simulink model "Quanser_AERO_Simulation_2020b"  (R2020b)
settings: Solver=ode45  StartTime=0.0  StopTime=2*sim_time  FixedStep=0.01  RelTol=1e-3
InitFcn:
  | % Run simulation parameters
  | quanser_AERO_sim_params;
model workspace (MAT data in the model file):
  a = Simulink.Parameter
  a.Value = 1.15
  a.DataType = 'auto'
  a.Dimensions = [1 1]
  a_a = Simulink.Parameter
  a_a.Value = 0.043381
  a_a.DataType = 'auto'
  a_a.Dimensions = [1 1]
  b = Simulink.Parameter
  b.Value = 0.2847
  b.DataType = 'auto'
  b.Dimensions = [1 1]
  b_b = Simulink.Parameter
  b_b.Value = 0.005
  b_b.DataType = 'auto'
  b_b.Dimensions = [1 1]
  c = Simulink.Parameter
  c.Value = 0.53573
  c.DataType = 'auto'
  c.Dimensions = [1 1]
  c_c = Simulink.Parameter
  c_c.Value = 0.005
  c_c.DataType = 'auto'
  c_c.Dimensions = [1 1]
  d = Simulink.Parameter
  d.Value = 0.0071058
  d.DataType = 'auto'
  d.Dimensions = [1 1]
  d_d = Simulink.Parameter
  d_d.Value = 0
  d_d.DataType = 'auto'
  d_d.Dimensions = [1 1]
  e = Simulink.Parameter
  e.Value = 0.0071
  e.DataType = 'auto'
  e.Dimensions = [1 1]
  f = Simulink.Parameter
  f.Value = 0.05
  f.DataType = 'auto'
  f.Dimensions = [1 1]
  g = Simulink.Parameter
  g.Value = 9.81
  g.DataType = 'auto'
  g.Dimensions = [1 1]
  p_p = Simulink.Parameter
  p_p.Value = 0.0005466
  p_p.DataType = 'auto'
  p_p.Dimensions = [1 1]
  smiData.RigidTransform(1).translation = [75 240 -4.4408920985e-15]
  smiData.RigidTransform(1).angle = 1.57079632679
  smiData.RigidTransform(1).axis = [5.55111512313e-17 1 5.55111512313e-17]
  smiData.RigidTransform(1).ID = 'B[AERO - Fork:1:-:AERO - Arm:1]'
  smiData.RigidTransform(2).translation = [0 0 72.5]
  smiData.RigidTransform(2).angle = 0
  smiData.RigidTransform(2).axis = [0 0 0]
  smiData.RigidTransform(2).ID = 'F[AERO - Fork:1:-:AERO - Arm:1]'
  smiData.RigidTransform(3).translation = [53 0 0]
  smiData.RigidTransform(3).angle = 1.57079632679
  smiData.RigidTransform(3).axis = [0 -1 0]
  smiData.RigidTransform(3).ID = 'B[AERO - Arm:1:-:AERO - Propeller Housing:1]'
  smiData.RigidTransform(4).translation = [-2.67952073108e-14 10 -95.5137103749]
  smiData.RigidTransform(4).angle = 3.14159265359
  smiData.RigidTransform(4).axis = [1 0 0]
  smiData.RigidTransform(4).ID = 'F[AERO - Arm:1:-:AERO - Propeller Housing:1]'
  smiData.RigidTransform(5).translation = [-53 0 0]
  smiData.RigidTransform(5).angle = 3.14159265359
  smiData.RigidTransform(5).axis = [0.707106781187 0 0.707106781187]
  smiData.RigidTransform(5).ID = 'B[AERO - Arm:1:-:AERO - Propeller Housing:2]'
  smiData.RigidTransform(6).translation = [-2.67952073108e-14 10 -95.5137103749]
  smiData.RigidTransform(6).angle = 3.14159265359
  smiData.RigidTransform(6).axis = [1 0 0]
  smiData.RigidTransform(6).ID = 'F[AERO - Arm:1:-:AERO - Propeller Housing:2]'
  smiData.RigidTransform(7).translation = [0 90 0]
  smiData.RigidTransform(7).angle = 2.09439510239
  smiData.RigidTransform(7).axis = [-0.57735026919 -0.57735026919 -0.57735026919]
  smiData.RigidTransform(7).ID = 'B[AERO - Base:1:-:AERO - Fork:1]'
  smiData.RigidTransform(8).translation = [0 -10 -1.83697019872e-15]
  smiData.RigidTransform(8).angle = 1.57079632679
  smiData.RigidTransform(8).axis = [-1 0 0]
  smiData.RigidTransform(8).ID = 'F[AERO - Base:1:-:AERO - Fork:1]'
  smiData.RigidTransform(9).translation = [0 7 0]
  smiData.RigidTransform(9).angle = 1.57079632679
  smiData.RigidTransform(9).axis = [-1 1.5327705937e-16 1.5327705937e-16]
  smiData.RigidTransform(9).ID = 'B[AERO - Propeller Housing:1:-:AERO - Propeller:1]'
  smiData.RigidTransform(10).translation = [0 2 0]
  smiData.RigidTransform(10).angle = 1.6664335536
  smiData.RigidTransform(10).axis = [-0.908660854566 0.295241808844 0.295241808844]
  smiData.RigidTransform(10).ID = 'F[AERO - Propeller Housing:1:-:AERO - Propeller:1]'
  smiData.RigidTransform(11).translation = [0 7 0]
  smiData.RigidTransform(11).angle = 1.57079632679
  smiData.RigidTransform(11).axis = [-1 6.25051204106e-17 6.25051204106e-17]
  smiData.RigidTransform(11).ID = 'B[AERO - Propeller Housing:2:-:AERO - Propeller:2]'
  smiData.RigidTransform(12).translation = [0 2 0]
  smiData.RigidTransform(12).angle = 2.28432867519
  smiData.RigidTransform(12).axis = [-0.456966311669 -0.628960169645 -0.628960169645]
  smiData.RigidTransform(12).ID = 'F[AERO - Propeller Housing:2:-:AERO - Propeller:2]'
  smiData.RigidTransform(13).translation = [-4.21383634609 -51.619496794 8.881784197e-15]
  smiData.RigidTransform(13).angle = 0
  smiData.RigidTransform(13).axis = [0 0 0]
  smiData.RigidTransform(13).ID = 'SixDofRigidTransform[AERO - Base:1]'
  smiData.Solid(1).mass = 2.36460135901
  smiData.Solid(1).CoM = [5.24111117378e-10 37.9532129776 0]
  smiData.Solid(1).MoI = [7187.732483 11870.3385044 7187.73246752]
  smiData.Solid(1).PoI = [0 0 -5.80827271444e-08]
  smiData.Solid(1).color = [0.0196078431373 0.0196078431373 0.0196078431373]
  smiData.Solid(1).opacity = 1
  smiData.Solid(1).ID = 'AERO - Base.ipt_{5B170AF7-4835-771C-6ADF-04BDBD784493}'
  smiData.Solid(2).mass = 0.833057949362
  smiData.Solid(2).CoM = [2.66169728603e-11 94.8876622043 1.47659785864e-12]
  smiData.Solid(2).MoI = [5303.1260885 5291.93963258 10383.1205417]
  smiData.Solid(2).PoI = [-1.78319566538e-10 1.20053300634e-10 2.21603950608e-09]
  smiData.Solid(2).color = [0.0196078431373 0.0196078431373 0.0196078431373]
  smiData.Solid(2).opacity = 1
  smiData.Solid(2).ID = 'AERO - Fork.ipt_{19DEB560-4DA8-F02E-E9C0-369FCF880C44}'
  smiData.Solid(3).mass = 0.268036846773
  smiData.Solid(3).CoM = [1.42171296006e-09 -5.19659809406e-10 0]
  smiData.Solid(3).MoI = [365.292105474 461.18513674 151.85502279]
  smiData.Solid(3).PoI = [9.09494701773e-14 -7.58518581279e-10 0]
  smiData.Solid(3).color = [0.0196078431373 0.0196078431373 0.0196078431373]
  smiData.Solid(3).opacity = 1
  smiData.Solid(3).ID = 'AERO - Arm.ipt_{15B1D815-460D-A329-2F9F-5FB9E93ED37B}'
  smiData.Solid(4).mass = 0.12383177107
  smiData.Solid(4).CoM = [0.00177195297055 5.45503898669 -8.60877968745]
  smiData.Solid(4).MoI = [310.701431452 411.715449483 138.600608927]
  smiData.Solid(4).PoI = [4.84491065682 -0.146839869659 -0.00100363322073]
  smiData.Solid(4).color = [0.0196078431373 0.0196078431373 0.0196078431373]
  smiData.Solid(4).opacity = 1
  smiData.Solid(4).ID = 'AERO - Propeller Housing.ipt_{180F9119-4C93-59E3-A88D-3BA97F46F3C3}'
  smiData.Solid(5).mass = 0.0206425497221
  smiData.Solid(5).CoM = [-1.0654070865e-12 5.09575570658 -2.10819251568e-11]
  smiData.Solid(5).MoI = [13.8216638961 27.2772869122 13.8216638974]
  smiData.Solid(5).PoI = [0 0 -9.39933149128e-14]
  smiData.Solid(5).color = [0.121568627451 0.121568627451 0.705882352941]
  smiData.Solid(5).opacity = 1
  smiData.Solid(5).ID = 'AERO - Propeller.ipt_{54ECD9B7-47A0-F6BB-CE8E-F5BB4731363E}'
  smiData.RevoluteJoint(1).Rz.Pos = 8.54433050095e-10
  smiData.RevoluteJoint(1).ID = '[AERO - Fork:1:-:AERO - Arm:1]'
  smiData.RevoluteJoint(2).Rz.Pos = 176.894023419
  smiData.RevoluteJoint(2).ID = '[AERO - Arm:1:-:AERO - Propeller Housing:1]'
  smiData.RevoluteJoint(3).Rz.Pos = 3.10597658118
  smiData.RevoluteJoint(3).ID = '[AERO - Arm:1:-:AERO - Propeller Housing:2]'
  smiData.RevoluteJoint(4).Rz.Pos = -4.73234748156e-11
  smiData.RevoluteJoint(4).ID = '[AERO - Base:1:-:AERO - Fork:1]'
  smiData.RevoluteJoint(5).Rz.Pos = -5.89066785065e-05
  smiData.RevoluteJoint(5).ID = '[AERO - Propeller Housing:1:-:AERO - Propeller:1]'
  smiData.RevoluteJoint(6).Rz.Pos = -3.64250166753e-05
  smiData.RevoluteJoint(6).ID = '[AERO - Propeller Housing:2:-:AERO - Propeller:2]'
  t_t = Simulink.Parameter
  t_t.Value = 0.0005466
  t_t.DataType = 'auto'
  t_t.Dimensions = [1 1]
  u_lim = Simulink.Parameter
  u_lim.Value = 24
  u_lim.DataType = 'auto'
  u_lim.Dimensions = [1 1]
  y_y = Simulink.Parameter
  y_y.Value = 0.02
  y_y.DataType = 'auto'
  y_y.Dimensions = [1 1]
  z_z = Simulink.Parameter
  z_z.Value = 0.01
  z_z.DataType = 'auto'
  z_z.Dimensions = [1 1]
values from neighbouring files (symbols this model uses):
  model = 1    [quanser_AERO_sim_params.m]
  ts = 0.002    [quanser_AERO_sim_params.m]
undefined symbols (not defined in the file or in its folder): delta, delta_a_range, delta_b_range, delta_c_range, den, dena, denb, dend, ini_cond, K, noise, num, numa, numb, numd, X, Y, Z
libraries: sm_lib x595, nesl_utility x119, simulink x102
(part 1 of 18)
settings Model: DataDictionary=AERO_DigitalTwin.sldd  OrderedModelArguments=off  Creator=garciar1  LastModifiedBy=linesLK
settings ExplorerConfigSet: InternalSimMechanicsExplorerSettings="<ExplorerConfiguration><canonicalview>planar_xy</canonicalview><AnimationSetting><BasePlaybackSpeed>1.0</BasePlaybackSpeed><PlaybackSpeedFactor>1.0</PlaybackSpeedFactor></AnimationSetting><TilePanel><TileInfo><Tiles Columns=\"1\" Count=\"1\" Rows=\"1\"><Column Weight=\"1\"/><Row Weight=\"1\"/><Tile Height=\"1\" Width=\"1\" X=\"0\" Y=\"0\"/></Tiles></TileInfo><SceneInfo><SceneViewer><BGColor><R>0.60000002384185791</R><G>0.60000002384185791</G><B>0.60000002384185791</B></BGColor><Camera><DoPerspective>off</DoPerspective><Position><X>0.606138610969192748</X><Y>0.738169372517540556</Y><Z>0.590514966088055981</Z></Position><Center><X>0.0287883417795668992</X><Y>0.160819103327914742</Y><Z>0.0131646968984300838</Z></Center><Up><X>-0.408248290463863073</X><Y>0.816496580927726145</Y><Z>-0.408248290463863073</Z></Up><ViewLimDist>1</ViewLimDist><YLim>0.238299283981323246</YLim><XLim>0.228027763120059318</XLim></Camera></SceneViewer></SceneInfo></TilePanel><MechEditorPanel><Cameras/><GfxPanelCameraMap/><VideoCreator><PlaybackSpeedRatio>1.0</PlaybackSpeedRatio><FrameRate>30</FrameRate><VideoFormat>Motion JPEG AVI</VideoFormat><FrameSize>auto</FrameSize></VideoCreator></MechEditorPanel></ExplorerConfiguration>"

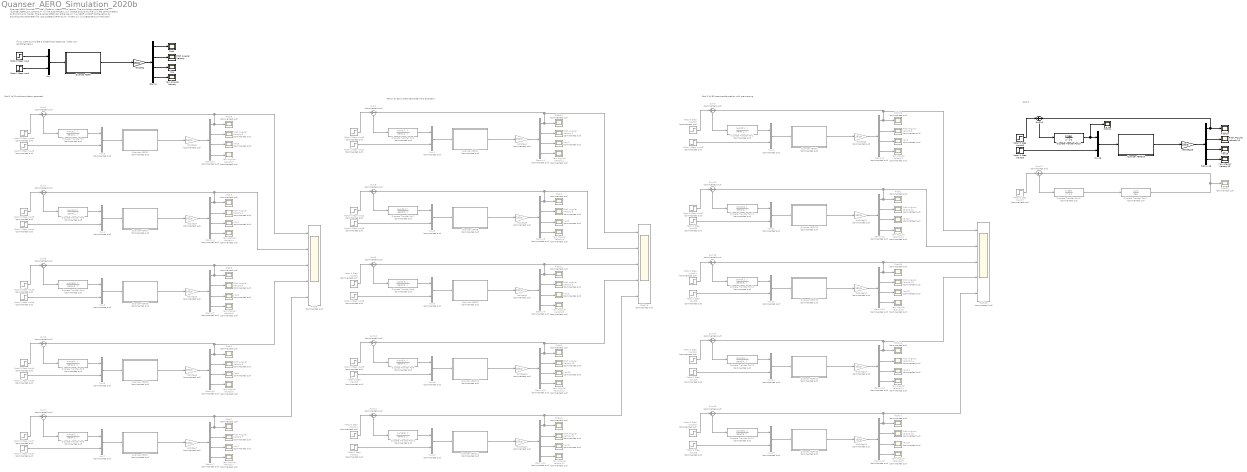
== system Quanser_AERO_Simulation_2020b ==
  note: If you want to simulate a closed-loop response, insert your controller below.
  note: Quanser AERO Simulation Model: Platform Independent Version
      | The simulation parameter file 'quanser_AERO_sim_params.m' will be automatically run, please ensure this file is in the same directory as this Simulink model. The Quanser AERO can either be run in a 1DOF or 2DOF configuration by adjusting the parameter file.
      | Last updated 29-07-21 by Vincent Liu (liuv2@student.unimelb.edu)
  note: Part 2 (a) Simple emulation approach
  note: Part 2 (b) Equivalent zero-order hold approach
  note: Part 2 (c) Bilinear transformation with pre-warping
  note: Part 3
  Demux : Demux
  Demux{1..15} (15 alike) : Demux  Commented=on
  Demux16 : Demux
  Discrete Transfer Fcn : DiscreteTransferFcn  Commented=on  Numerator=numa(1, :)  Denominator=dena(1, :)  SampleTime=delta_a_range(1)
  Discrete Transfer Fcn1 : DiscreteTransferFcn  Commented=on  Numerator=numb(1, :)  Denominator=denb(1, :)  SampleTime=delta_b_range(1)
  Discrete Transfer Fcn10 : DiscreteTransferFcn  Commented=on  Numerator=numb(5, :)  Denominator=denb(5, :)  SampleTime=delta_b_range(5)
  Discrete Transfer Fcn11 : DiscreteTransferFcn  Commented=on  Numerator=numd(2,:)  Denominator=dend(2,:)  SampleTime=delta_c_range(2)
  Discrete Transfer Fcn12 : DiscreteTransferFcn  Commented=on  Numerator=numd(3, :)  Denominator=dend(3, :)  SampleTime=delta_c_range(3)
  Discrete Transfer Fcn13 : DiscreteTransferFcn  Commented=on  Numerator=numd(4, :)  Denominator=dend(4, :)  SampleTime=delta_c_range(4)
  Discrete Transfer Fcn14 : DiscreteTransferFcn  Commented=on  Numerator=numd(5, :)  Denominator=dend(5, :)  SampleTime=delta_c_range(5)
  Discrete Transfer Fcn15 : DiscreteTransferFcn  Numerator=K*den  Denominator=[1 -1 0]  SampleTime=delta
  Discrete Transfer Fcn16 : DiscreteTransferFcn  Commented=on  Numerator=K*den  Denominator=[1 -1 0]  SampleTime=delta
  Discrete Transfer Fcn17 : DiscreteTransferFcn  Commented=on  Numerator=num  Denominator=den  SampleTime=delta
  Discrete Transfer Fcn2 : DiscreteTransferFcn  Commented=on  Numerator=numd(1, :)  Denominator=dend(1, :)  SampleTime=delta_c_range(1)
  Discrete Transfer Fcn3 : DiscreteTransferFcn  Commented=on  Numerator=numa(2,:)  Denominator=dena(2,:)  SampleTime=delta_a_range(2)
  Discrete Transfer Fcn4 : DiscreteTransferFcn  Commented=on  Numerator=numa(3, :)  Denominator=dena(3, :)  SampleTime=delta_a_range(3)
  Discrete Transfer Fcn5 : DiscreteTransferFcn  Commented=on  Numerator=numa(4, :)  Denominator=dena(4, :)  SampleTime=delta_a_range(4)
  Discrete Transfer Fcn6 : DiscreteTransferFcn  Commented=on  Numerator=numa(5, :)  Denominator=dena(5, :)  SampleTime=delta_a_range(5)
  Discrete Transfer Fcn7 : DiscreteTransferFcn  Commented=on  Numerator=numb(2,:)  Denominator=denb(2,:)  SampleTime=delta_b_range(2)
  Discrete Transfer Fcn8 : DiscreteTransferFcn  Commented=on  Numerator=numb(3, :)  Denominator=denb(3, :)  SampleTime=delta_b_range(3)
  Discrete Transfer Fcn9 : DiscreteTransferFcn  Commented=on  Numerator=numb(4, :)  Denominator=denb(4, :)  SampleTime=delta_b_range(4)
  Motor 0 Step Input : Step  After=20  SampleTime=0
  Motor 0 Step Input{1..15,17} (16 alike) : Step  Commented=on  After=10  SampleTime=0
  Motor 0 Step Input16 : Step  After=10  SampleTime=0
  Motor 1 Step Input : Step  After=10  SampleTime=0
  Motor 1 Step Input{1..15} (15 alike) : Step  Commented=on  After=10  SampleTime=0
  Motor 1 Step Input16 : Step  After=10  SampleTime=0
  Mux : Mux  Inputs=2
  Mux{1..15} (15 alike) : Mux  Commented=on  Inputs=2
  Mux16 : Mux  Inputs=2
  Pitch : Scope
  Pitch Angular Velocity : Scope
  Pitch Angular Velocity{1..15} (15 alike) : Scope  Commented=on
  Pitch Angular Velocity16 : Scope
  Pitch{1..7,9..12,14..17,20} (16 alike) : Scope  Commented=on
  Pitch13 : Scope  Commented=on  NumInputPorts=5
  Pitch18 : Scope  Commented=on  NumInputPorts=5
  Pitch19 : Scope
  Pitch21 : Scope
  Pitch8 : Scope  Commented=on  NumInputPorts=5
  Quanser AERO : Subsystem  TreatAsAtomicUnit=on
  Quanser AERO1 : Subsystem  Commented=on  TreatAsAtomicUnit=on
  Quanser AERO10 : Subsystem  Commented=on  TreatAsAtomicUnit=on
  Quanser AERO11 : Subsystem  Commented=on  TreatAsAtomicUnit=on
  Quanser AERO12 : Subsystem  Commented=on  TreatAsAtomicUnit=on
  Quanser AERO13 : Subsystem  Commented=on  TreatAsAtomicUnit=on
  Quanser AERO14 : Subsystem  Commented=on  TreatAsAtomicUnit=on
  Quanser AERO15 : Subsystem  Commented=on  TreatAsAtomicUnit=on
  Quanser AERO16 : Subsystem  TreatAsAtomicUnit=on
  Quanser AERO2 : Subsystem  Commented=on  TreatAsAtomicUnit=on
  Quanser AERO3 : Subsystem  Commented=on  TreatAsAtomicUnit=on
  Quanser AERO4 : Subsystem  Commented=on  TreatAsAtomicUnit=on
  Quanser AERO5 : Subsystem  Commented=on  TreatAsAtomicUnit=on
  Quanser AERO6 : Subsystem  Commented=on  TreatAsAtomicUnit=on
  Quanser AERO7 : Subsystem  Commented=on  TreatAsAtomicUnit=on
  Quanser AERO8 : Subsystem  Commented=on  TreatAsAtomicUnit=on
  Quanser AERO9 : Subsystem  Commented=on  TreatAsAtomicUnit=on
  Sum{1..15,17} (16 alike) : Sum  Commented=on  Inputs=+-
  Sum16 : Sum  Inputs=+-
  Yaw : Scope
  Yaw Angular Velocity : Scope
  Yaw Angular Velocity{1..15} (15 alike) : Scope  Commented=on
  Yaw Angular Velocity16 : Scope
  Yaw{1..15} (15 alike) : Scope  Commented=on
  Yaw16 : Scope
  rad2deg : Gain  Gain=180/pi
  rad2deg{1..15} (15 alike) : Gain  Commented=on  Gain=180/pi
  rad2deg16 : Gain  Gain=180/pi
  wires:
  Demux/3 -> Yaw/1
  Demux/2 -> Pitch Angular Velocity/1
  Demux/4 -> Yaw Angular Velocity/1
  Mux/1 -> Quanser AERO/1(u)  "[V0; V1]"
  rad2deg/1 -> Demux/1
  Quanser AERO/1(x) -> rad2deg/1  "[theta; theta_d; psi; psi_d]"
  Motor 1 Step Input/1 -> Mux/2
  Motor 0 Step Input/1 -> Mux/1
  Demux/1 -> Pitch/1
  rad2deg2/1 -> Demux3/1
  Demux3/1 -> Pitch5/1, Pitch8/1, Sum2/2  "Delta = 0.045"
  Demux3/4 -> Yaw Angular Velocity3/1
  Demux3/3 -> Yaw3/1
  Demux3/2 -> Pitch Angular Velocity3/1
  Motor 1 Step Input3/1 -> Mux3/2
  Quanser AERO3/1(x) -> rad2deg2/1  "[theta; theta_d; psi; psi_d]"
  Mux3/1 -> Quanser AERO3/1(u)  "[V0; V1]"
  Discrete Transfer Fcn/1 -> Mux3/1
  Motor 0 Step Input5/1 -> Sum2/1
  Sum2/1 -> Discrete Transfer Fcn/1
  Mux4/1 -> Quanser AERO4/1(u)  "[V0; V1]"
  Demux4/3 -> Yaw4/1
  Quanser AERO4/1(x) -> rad2deg4/1  "[theta; theta_d; psi; psi_d]"
  Motor 1 Step Input4/1 -> Mux4/2
  Demux4/1 -> Pitch8/2, Sum4/2, Pitch3/1  "Delta = 0.0475"
  rad2deg4/1 -> Demux4/1
  Sum4/1 -> Discrete Transfer Fcn3/1
  Demux4/4 -> Yaw Angular Velocity4/1
  Demux4/2 -> Pitch Angular Velocity4/1
  Motor 0 Step Input3/1 -> Sum4/1
  Discrete Transfer Fcn3/1 -> Mux4/1
  Demux5/3 -> Yaw5/1
  Sum6/1 -> Discrete Transfer Fcn5/1
  Demux6/3 -> Yaw6/1
  rad2deg5/1 -> Demux5/1
  Mux5/1 -> Quanser AERO5/1(u)  "[V0; V1]"
  Motor 0 Step Input4/1 -> Sum6/1
  Quanser AERO5/1(x) -> rad2deg5/1  "[theta; theta_d; psi; psi_d]"
  Demux5/2 -> Pitch Angular Velocity5/1
  Motor 0 Step Input6/1 -> Sum5/1
  Demux5/4 -> Yaw Angular Velocity5/1
  Discrete Transfer Fcn4/1 -> Mux5/1
  Motor 1 Step Input6/1 -> Mux6/2
  Demux5/1 -> Pitch6/1, Sum5/2, Pitch8/3  "Delta = 0.05"
  Sum5/1 -> Discrete Transfer Fcn4/1
  Mux6/1 -> Quanser AERO6/1(u)  "[V0; V1]"
  Quanser AERO6/1(x) -> rad2deg6/1  "[theta; theta_d; psi; psi_d]"
  Motor 1 Step Input5/1 -> Mux5/2
  Demux6/2 -> Pitch Angular Velocity6/1
  Demux6/4 -> Yaw Angular Velocity6/1
  Discrete Transfer Fcn5/1 -> Mux6/1
  rad2deg6/1 -> Demux6/1
  Demux6/1 -> Pitch4/1, Pitch8/4, Sum6/2  "Delta = 0.0525"
  Mux7/1 -> Quanser AERO7/1(u)  "[V0; V1]"
  Motor 1 Step Input7/1 -> Mux7/2
  rad2deg7/1 -> Demux7/1
  Demux7/4 -> Yaw Angular Velocity7/1
  Demux7/3 -> Yaw7/1
  Motor 0 Step Input7/1 -> Sum7/1
  Discrete Transfer Fcn6/1 -> Mux7/1
  Quanser AERO7/1(x) -> rad2deg7/1  "[theta; theta_d; psi; psi_d]"
  Demux7/2 -> Pitch Angular Velocity7/1
  Sum7/1 -> Discrete Transfer Fcn6/1
  Demux7/1 -> Pitch7/1, Pitch8/5, Sum7/2  "Delta = 0.055"
  Motor 1 Step Input10/1 -> Mux10/2
  Demux11/1 -> Pitch12/1, Pitch13/5, Sum11/2  "Delta = 0.0475"
  Demux1/4 -> Yaw Angular Velocity1/1
  Demux10/4 -> Yaw Angular Velocity10/1
  rad2deg11/1 -> Demux11/1
  rad2deg8/1 -> Demux8/1
  Demux8/4 -> Yaw Angular Velocity8/1
  Discrete Transfer Fcn8/1 -> Mux9/1
  Demux11/2 -> Pitch Angular Velocity11/1
  Motor 0 Step Input11/1 -> Sum11/1
  Demux10/2 -> Pitch Angular Velocity10/1
  Mux10/1 -> Quanser AERO10/1(u)  "[V0; V1]"
  rad2deg9/1 -> Demux9/1
  Discrete Transfer Fcn9/1 -> Mux10/1
  Sum11/1 -> Discrete Transfer Fcn10/1
  Quanser AERO1/1(x) -> rad2deg1/1  "[theta; theta_d; psi; psi_d]"
  Motor 1 Step Input1/1 -> Mux1/2
  Discrete Transfer Fcn7/1 -> Mux8/1
  Demux8/1 -> Pitch13/2, Sum8/2, Pitch1/1  "Delta = 0.04"
  Demux1/3 -> Yaw1/1
  Motor 1 Step Input11/1 -> Mux11/2
  Demux10/1 -> Pitch9/1, Pitch13/4, Sum10/2  "Delta = 0.045"
  Demux9/3 -> Yaw9/1
  Motor 0 Step Input8/1 -> Sum10/1
  Sum9/1 -> Discrete Transfer Fcn8/1
  Sum1/1 -> Discrete Transfer Fcn1/1
  Motor 0 Step Input9/1 -> Sum1/1
  Sum8/1 -> Discrete Transfer Fcn7/1
  Motor 1 Step Input9/1 -> Mux9/2
  Demux1/2 -> Pitch Angular Velocity1/1
  Discrete Transfer Fcn1/1 -> Mux1/1
  Quanser AERO9/1(x) -> rad2deg9/1  "[theta; theta_d; psi; psi_d]"
  Mux1/1 -> Quanser AERO1/1(u)  "[V0; V1]"
  Mux8/1 -> Quanser AERO8/1(u)  "[V0; V1]"
  Quanser AERO8/1(x) -> rad2deg8/1  "[theta; theta_d; psi; psi_d]"
  Demux8/2 -> Pitch Angular Velocity8/1
  Demux1/1 -> Pitch10/1, Pitch13/1, Sum1/2  "Delta = 0.0375"
  Motor 1 Step Input8/1 -> Mux8/2
  Demux9/2 -> Pitch Angular Velocity9/1
  Demux9/4 -> Yaw Angular Velocity9/1
  Motor 0 Step Input10/1 -> Sum9/1
  Mux9/1 -> Quanser AERO9/1(u)  "[V0; V1]"
  Demux9/1 -> Pitch11/1, Sum9/2, Pitch13/3  "Delta = 0.0425"
  Demux8/3 -> Yaw8/1
  Demux11/4 -> Yaw Angular Velocity11/1
  Motor 0 Step Input1/1 -> Sum8/1
  Discrete Transfer Fcn10/1 -> Mux11/1
  Demux11/3 -> Yaw11/1
  rad2deg1/1 -> Demux1/1
  rad2deg10/1 -> Demux10/1
  Demux10/3 -> Yaw10/1
  Mux11/1 -> Quanser AERO11/1(u)  "[V0; V1]"
  Quanser AERO10/1(x) -> rad2deg10/1  "[theta; theta_d; psi; psi_d]"
  Sum10/1 -> Discrete Transfer Fcn9/1
  Quanser AERO11/1(x) -> rad2deg11/1  "[theta; theta_d; psi; psi_d]"
  Motor 1 Step Input14/1 -> Mux14/2
  Demux15/1 -> Pitch17/1, Pitch18/5, Sum15/2  "Delta = 0.055"
  Demux2/4 -> Yaw Angular Velocity2/1
  Demux14/4 -> Yaw Angular Velocity14/1
  rad2deg15/1 -> Demux15/1
  rad2deg12/1 -> Demux12/1
  Demux12/4 -> Yaw Angular Velocity12/1
  Discrete Transfer Fcn12/1 -> Mux13/1
  Demux15/2 -> Pitch Angular Velocity15/1
  Motor 0 Step Input15/1 -> Sum15/1
  Demux14/2 -> Pitch Angular Velocity14/1
  Mux14/1 -> Quanser AERO14/1(u)  "[V0; V1]"
  rad2deg13/1 -> Demux13/1
  Discrete Transfer Fcn13/1 -> Mux14/1
  Sum15/1 -> Discrete Transfer Fcn14/1
  Quanser AERO2/1(x) -> rad2deg3/1  "[theta; theta_d; psi; psi_d]"
  Motor 1 Step Input2/1 -> Mux2/2
  Discrete Transfer Fcn11/1 -> Mux12/1
  Demux12/1 -> Pitch18/2, Sum12/2, Pitch2/1  "Delta = 0.0475"
  Demux2/3 -> Yaw2/1
  Motor 1 Step Input15/1 -> Mux15/2
  Demux14/1 -> Pitch14/1, Pitch18/4, Sum14/2  "Delta = 0.0525"
  Demux13/3 -> Yaw13/1
  Motor 0 Step Input12/1 -> Sum14/1
  Sum13/1 -> Discrete Transfer Fcn12/1
  Sum3/1 -> Discrete Transfer Fcn2/1
  Motor 0 Step Input13/1 -> Sum3/1
  Sum12/1 -> Discrete Transfer Fcn11/1
  Motor 1 Step Input13/1 -> Mux13/2
  Demux2/2 -> Pitch Angular Velocity2/1
  Discrete Transfer Fcn2/1 -> Mux2/1
  Quanser AERO13/1(x) -> rad2deg13/1  "[theta; theta_d; psi; psi_d]"
  Mux2/1 -> Quanser AERO2/1(u)  "[V0; V1]"
  Mux12/1 -> Quanser AERO12/1(u)  "[V0; V1]"
  Quanser AERO12/1(x) -> rad2deg12/1  "[theta; theta_d; psi; psi_d]"
  Demux12/2 -> Pitch Angular Velocity12/1
  Demux2/1 -> Pitch15/1, Pitch18/1, Sum3/2  "Delta = 0.045"
  Motor 1 Step Input12/1 -> Mux12/2
  Demux13/2 -> Pitch Angular Velocity13/1
  Demux13/4 -> Yaw Angular Velocity13/1
  Motor 0 Step Input14/1 -> Sum13/1
  Mux13/1 -> Quanser AERO13/1(u)  "[V0; V1]"
  Demux13/1 -> Pitch16/1, Sum13/2, Pitch18/3  "Delta = 0.05"
  Demux12/3 -> Yaw12/1
  Demux15/4 -> Yaw Angular Velocity15/1
  Motor 0 Step Input2/1 -> Sum12/1
  Discrete Transfer Fcn14/1 -> Mux15/1
  Demux15/3 -> Yaw15/1
  rad2deg3/1 -> Demux2/1
  rad2deg14/1 -> Demux14/1
  Demux14/3 -> Yaw14/1
  Mux15/1 -> Quanser AERO15/1(u)  "[V0; V1]"
  Quanser AERO14/1(x) -> rad2deg14/1  "[theta; theta_d; psi; psi_d]"
  Sum14/1 -> Discrete Transfer Fcn13/1
  Quanser AERO15/1(x) -> rad2deg15/1  "[theta; theta_d; psi; psi_d]"
  rad2deg16/1 -> Demux16/1
  Sum16/1 -> Discrete Transfer Fcn15/1
  Motor 1 Step Input16/1 -> Mux16/2
  Quanser AERO16/1(x) -> rad2deg16/1  "[theta; theta_d; psi; psi_d]"
  Motor 0 Step Input16/1 -> Sum16/1
  Mux16/1 -> Quanser AERO16/1(u)  "[V0; V1]"
  Demux16/2 -> Pitch Angular Velocity16/1
  Discrete Transfer Fcn15/1 -> Pitch21/1, Mux16/1
  Demux16/3 -> Yaw16/1
  Demux16/1 -> Pitch19/1, Sum16/2  "Delta = 0.05"
  Demux16/4 -> Yaw Angular Velocity16/1
  Sum17/1 -> Discrete Transfer Fcn16/1
  Motor 0 Step Input17/1 -> Sum17/1
  Discrete Transfer Fcn16/1 -> Discrete Transfer Fcn17/1
  Discrete Transfer Fcn17/1 -> Pitch20/1, Sum17/2  "Delta = 0.05"

== system Quanser_AERO_Simulation_2020b/Quanser AERO ==
  u : Inport
  Constant : Constant  Value=model
  Demux : Demux  Outputs=2
  Demux1 : Demux  Outputs=2
  Digital Twin : Subsystem
  Input Noise : Subsystem  TreatAsAtomicUnit=on
  Integrator : Integrator  InitialCondition=[ini_cond.theta; ini_cond.theta_dot; ini_cond.psi; ini_cond.psi_dot]
  Measurement Noise : Subsystem  TreatAsAtomicUnit=on
  Quanser AERO System Dynamics : Subsystem  TreatAsAtomicUnit=on
  Rate Transition : RateTransition  OutPortSampleTime=ts
  Rate Transition1 : RateTransition  InitialCondition=[ini_cond.theta; ini_cond.theta_dot; ini_cond.psi; ini_cond.psi_dot]  OutPortSampleTime=ts
  Selector : Selector  InputPortWidth=4  IndexOptions=Index vector (dialog)  Indices=[1 3]  OutputSizes=1
  x : Outport  VectorParamsAs1DForOutWhenUnconnected=off
  wires:
  u/1 -> Rate Transition/1
  Rate Transition/1 -> Input Noise/1(u), Demux/1
  Rate Transition1/1 -> x/1
  Input Noise/1(u_noise) -> Quanser AERO System Dynamics/2(u)
  Measurement Noise/1(x_noise) -> Rate Transition1/1
  Selector/1 -> Demux1/1
  Demux/1 -> Digital Twin/3(thruster_1)
  Demux/2 -> Digital Twin/4(thruster_2)
  Demux1/1 -> Digital Twin/1(theta)
  Demux1/2 -> Digital Twin/2(psi)
  Integrator/1 -> Measurement Noise/1(x), Selector/1, Quanser AERO System Dynamics/1(x)
  Constant/1 -> Quanser AERO System Dynamics/3(model)
  Quanser AERO System Dynamics/1(x_dot) -> Integrator/1

== system Quanser_AERO_Simulation_2020b/Quanser AERO1 ==
  u : Inport
  Constant : Constant  Value=model
  Demux : Demux  Outputs=2
  Demux1 : Demux  Outputs=2
  Digital Twin : Subsystem
  Input Noise : Subsystem  TreatAsAtomicUnit=on
  Integrator : Integrator  InitialCondition=[ini_cond.theta; ini_cond.theta_dot; ini_cond.psi; ini_cond.psi_dot]
  Measurement Noise : Subsystem  TreatAsAtomicUnit=on
  Quanser AERO System Dynamics : Subsystem  TreatAsAtomicUnit=on
  Rate Transition : RateTransition  OutPortSampleTime=ts
  Rate Transition1 : RateTransition  InitialCondition=[ini_cond.theta; ini_cond.theta_dot; ini_cond.psi; ini_cond.psi_dot]  OutPortSampleTime=ts
  Selector : Selector  InputPortWidth=4  IndexOptions=Index vector (dialog)  Indices=[1 3]  OutputSizes=1
  x : Outport  VectorParamsAs1DForOutWhenUnconnected=off
  wires:
  u/1 -> Rate Transition/1
  Rate Transition/1 -> Input Noise/1(u), Demux/1
  Rate Transition1/1 -> x/1
  Input Noise/1(u_noise) -> Quanser AERO System Dynamics/2(u)
  Measurement Noise/1(x_noise) -> Rate Transition1/1
  Selector/1 -> Demux1/1
  Demux/1 -> Digital Twin/3(thruster_1)
  Demux/2 -> Digital Twin/4(thruster_2)
  Demux1/1 -> Digital Twin/1(theta)
  Demux1/2 -> Digital Twin/2(psi)
  Integrator/1 -> Measurement Noise/1(x), Selector/1, Quanser AERO System Dynamics/1(x)
  Constant/1 -> Quanser AERO System Dynamics/3(model)
  Quanser AERO System Dynamics/1(x_dot) -> Integrator/1

== system Quanser_AERO_Simulation_2020b/Quanser AERO10 ==
  u : Inport
  Constant : Constant  Value=model
  Demux : Demux  Outputs=2
  Demux1 : Demux  Outputs=2
  Digital Twin : Subsystem
  Input Noise : Subsystem  TreatAsAtomicUnit=on
  Integrator : Integrator  InitialCondition=[ini_cond.theta; ini_cond.theta_dot; ini_cond.psi; ini_cond.psi_dot]
  Measurement Noise : Subsystem  TreatAsAtomicUnit=on
  Quanser AERO System Dynamics : Subsystem  TreatAsAtomicUnit=on
  Rate Transition : RateTransition  OutPortSampleTime=ts
  Rate Transition1 : RateTransition  InitialCondition=[ini_cond.theta; ini_cond.theta_dot; ini_cond.psi; ini_cond.psi_dot]  OutPortSampleTime=ts
  Selector : Selector  InputPortWidth=4  IndexOptions=Index vector (dialog)  Indices=[1 3]  OutputSizes=1
  x : Outport  VectorParamsAs1DForOutWhenUnconnected=off
  wires:
  u/1 -> Rate Transition/1
  Rate Transition/1 -> Input Noise/1(u), Demux/1
  Rate Transition1/1 -> x/1
  Input Noise/1(u_noise) -> Quanser AERO System Dynamics/2(u)
  Measurement Noise/1(x_noise) -> Rate Transition1/1
  Selector/1 -> Demux1/1
  Demux/1 -> Digital Twin/3(thruster_1)
  Demux/2 -> Digital Twin/4(thruster_2)
  Demux1/1 -> Digital Twin/1(theta)
  Demux1/2 -> Digital Twin/2(psi)
  Integrator/1 -> Measurement Noise/1(x), Selector/1, Quanser AERO System Dynamics/1(x)
  Constant/1 -> Quanser AERO System Dynamics/3(model)
  Quanser AERO System Dynamics/1(x_dot) -> Integrator/1

== system Quanser_AERO_Simulation_2020b/Quanser AERO11 ==
  u : Inport
  Constant : Constant  Value=model
  Demux : Demux  Outputs=2
  Demux1 : Demux  Outputs=2
  Digital Twin : Subsystem
  Input Noise : Subsystem  TreatAsAtomicUnit=on
  Integrator : Integrator  InitialCondition=[ini_cond.theta; ini_cond.theta_dot; ini_cond.psi; ini_cond.psi_dot]
  Measurement Noise : Subsystem  TreatAsAtomicUnit=on
  Quanser AERO System Dynamics : Subsystem  TreatAsAtomicUnit=on
  Rate Transition : RateTransition  OutPortSampleTime=ts
  Rate Transition1 : RateTransition  InitialCondition=[ini_cond.theta; ini_cond.theta_dot; ini_cond.psi; ini_cond.psi_dot]  OutPortSampleTime=ts
  Selector : Selector  InputPortWidth=4  IndexOptions=Index vector (dialog)  Indices=[1 3]  OutputSizes=1
  x : Outport  VectorParamsAs1DForOutWhenUnconnected=off
  wires:
  u/1 -> Rate Transition/1
  Rate Transition/1 -> Input Noise/1(u), Demux/1
  Rate Transition1/1 -> x/1
  Input Noise/1(u_noise) -> Quanser AERO System Dynamics/2(u)
  Measurement Noise/1(x_noise) -> Rate Transition1/1
  Selector/1 -> Demux1/1
  Demux/1 -> Digital Twin/3(thruster_1)
  Demux/2 -> Digital Twin/4(thruster_2)
  Demux1/1 -> Digital Twin/1(theta)
  Demux1/2 -> Digital Twin/2(psi)
  Integrator/1 -> Measurement Noise/1(x), Selector/1, Quanser AERO System Dynamics/1(x)
  Constant/1 -> Quanser AERO System Dynamics/3(model)
  Quanser AERO System Dynamics/1(x_dot) -> Integrator/1

== system Quanser_AERO_Simulation_2020b/Quanser AERO12 ==
  u : Inport
  Constant : Constant  Value=model
  Demux : Demux  Outputs=2
  Demux1 : Demux  Outputs=2
  Digital Twin : Subsystem
  Input Noise : Subsystem  TreatAsAtomicUnit=on
  Integrator : Integrator  InitialCondition=[ini_cond.theta; ini_cond.theta_dot; ini_cond.psi; ini_cond.psi_dot]
  Measurement Noise : Subsystem  TreatAsAtomicUnit=on
  Quanser AERO System Dynamics : Subsystem  TreatAsAtomicUnit=on
  Rate Transition : RateTransition  OutPortSampleTime=ts
  Rate Transition1 : RateTransition  InitialCondition=[ini_cond.theta; ini_cond.theta_dot; ini_cond.psi; ini_cond.psi_dot]  OutPortSampleTime=ts
  Selector : Selector  InputPortWidth=4  IndexOptions=Index vector (dialog)  Indices=[1 3]  OutputSizes=1
  x : Outport  VectorParamsAs1DForOutWhenUnconnected=off
  wires:
  u/1 -> Rate Transition/1
  Rate Transition/1 -> Input Noise/1(u), Demux/1
  Rate Transition1/1 -> x/1
  Input Noise/1(u_noise) -> Quanser AERO System Dynamics/2(u)
  Measurement Noise/1(x_noise) -> Rate Transition1/1
  Selector/1 -> Demux1/1
  Demux/1 -> Digital Twin/3(thruster_1)
  Demux/2 -> Digital Twin/4(thruster_2)
  Demux1/1 -> Digital Twin/1(theta)
  Demux1/2 -> Digital Twin/2(psi)
  Integrator/1 -> Measurement Noise/1(x), Selector/1, Quanser AERO System Dynamics/1(x)
  Constant/1 -> Quanser AERO System Dynamics/3(model)
  Quanser AERO System Dynamics/1(x_dot) -> Integrator/1

== system Quanser_AERO_Simulation_2020b/Quanser AERO13 ==
  u : Inport
  Constant : Constant  Value=model
  Demux : Demux  Outputs=2
  Demux1 : Demux  Outputs=2
  Digital Twin : Subsystem
  Input Noise : Subsystem  TreatAsAtomicUnit=on
  Integrator : Integrator  InitialCondition=[ini_cond.theta; ini_cond.theta_dot; ini_cond.psi; ini_cond.psi_dot]
  Measurement Noise : Subsystem  TreatAsAtomicUnit=on
  Quanser AERO System Dynamics : Subsystem  TreatAsAtomicUnit=on
  Rate Transition : RateTransition  OutPortSampleTime=ts
  Rate Transition1 : RateTransition  InitialCondition=[ini_cond.theta; ini_cond.theta_dot; ini_cond.psi; ini_cond.psi_dot]  OutPortSampleTime=ts
  Selector : Selector  InputPortWidth=4  IndexOptions=Index vector (dialog)  Indices=[1 3]  OutputSizes=1
  x : Outport  VectorParamsAs1DForOutWhenUnconnected=off
  wires:
  u/1 -> Rate Transition/1
  Rate Transition/1 -> Input Noise/1(u), Demux/1
  Rate Transition1/1 -> x/1
  Input Noise/1(u_noise) -> Quanser AERO System Dynamics/2(u)
  Measurement Noise/1(x_noise) -> Rate Transition1/1
  Selector/1 -> Demux1/1
  Demux/1 -> Digital Twin/3(thruster_1)
  Demux/2 -> Digital Twin/4(thruster_2)
  Demux1/1 -> Digital Twin/1(theta)
  Demux1/2 -> Digital Twin/2(psi)
  Integrator/1 -> Measurement Noise/1(x), Selector/1, Quanser AERO System Dynamics/1(x)
  Constant/1 -> Quanser AERO System Dynamics/3(model)
  Quanser AERO System Dynamics/1(x_dot) -> Integrator/1

== system Quanser_AERO_Simulation_2020b/Quanser AERO14 ==
  u : Inport
  Constant : Constant  Value=model
  Demux : Demux  Outputs=2
  Demux1 : Demux  Outputs=2
  Digital Twin : Subsystem
  Input Noise : Subsystem  TreatAsAtomicUnit=on
  Integrator : Integrator  InitialCondition=[ini_cond.theta; ini_cond.theta_dot; ini_cond.psi; ini_cond.psi_dot]
  Measurement Noise : Subsystem  TreatAsAtomicUnit=on
  Quanser AERO System Dynamics : Subsystem  TreatAsAtomicUnit=on
  Rate Transition : RateTransition  OutPortSampleTime=ts
  Rate Transition1 : RateTransition  InitialCondition=[ini_cond.theta; ini_cond.theta_dot; ini_cond.psi; ini_cond.psi_dot]  OutPortSampleTime=ts
  Selector : Selector  InputPortWidth=4  IndexOptions=Index vector (dialog)  Indices=[1 3]  OutputSizes=1
  x : Outport  VectorParamsAs1DForOutWhenUnconnected=off
  wires:
  u/1 -> Rate Transition/1
  Rate Transition/1 -> Input Noise/1(u), Demux/1
  Rate Transition1/1 -> x/1
  Input Noise/1(u_noise) -> Quanser AERO System Dynamics/2(u)
  Measurement Noise/1(x_noise) -> Rate Transition1/1
  Selector/1 -> Demux1/1
  Demux/1 -> Digital Twin/3(thruster_1)
  Demux/2 -> Digital Twin/4(thruster_2)
  Demux1/1 -> Digital Twin/1(theta)
  Demux1/2 -> Digital Twin/2(psi)
  Integrator/1 -> Measurement Noise/1(x), Selector/1, Quanser AERO System Dynamics/1(x)
  Constant/1 -> Quanser AERO System Dynamics/3(model)
  Quanser AERO System Dynamics/1(x_dot) -> Integrator/1

== system Quanser_AERO_Simulation_2020b/Quanser AERO15 ==
  u : Inport
  Constant : Constant  Value=model
  Demux : Demux  Outputs=2
  Demux1 : Demux  Outputs=2
  Digital Twin : Subsystem
  Input Noise : Subsystem  TreatAsAtomicUnit=on
  Integrator : Integrator  InitialCondition=[ini_cond.theta; ini_cond.theta_dot; ini_cond.psi; ini_cond.psi_dot]
  Measurement Noise : Subsystem  TreatAsAtomicUnit=on
  Quanser AERO System Dynamics : Subsystem  TreatAsAtomicUnit=on
  Rate Transition : RateTransition  OutPortSampleTime=ts
  Rate Transition1 : RateTransition  InitialCondition=[ini_cond.theta; ini_cond.theta_dot; ini_cond.psi; ini_cond.psi_dot]  OutPortSampleTime=ts
  Selector : Selector  InputPortWidth=4  IndexOptions=Index vector (dialog)  Indices=[1 3]  OutputSizes=1
  x : Outport  VectorParamsAs1DForOutWhenUnconnected=off
  wires:
  u/1 -> Rate Transition/1
  Rate Transition/1 -> Input Noise/1(u), Demux/1
  Rate Transition1/1 -> x/1
  Input Noise/1(u_noise) -> Quanser AERO System Dynamics/2(u)
  Measurement Noise/1(x_noise) -> Rate Transition1/1
  Selector/1 -> Demux1/1
  Demux/1 -> Digital Twin/3(thruster_1)
  Demux/2 -> Digital Twin/4(thruster_2)
  Demux1/1 -> Digital Twin/1(theta)
  Demux1/2 -> Digital Twin/2(psi)
  Integrator/1 -> Measurement Noise/1(x), Selector/1, Quanser AERO System Dynamics/1(x)
  Constant/1 -> Quanser AERO System Dynamics/3(model)
  Quanser AERO System Dynamics/1(x_dot) -> Integrator/1

== system Quanser_AERO_Simulation_2020b/Quanser AERO16 ==
  u : Inport
  Constant : Constant  Value=model
  Demux : Demux  Outputs=2
  Demux1 : Demux  Outputs=2
  Digital Twin : Subsystem
  Input Noise : Subsystem  TreatAsAtomicUnit=on
  Integrator : Integrator  InitialCondition=[ini_cond.theta; ini_cond.theta_dot; ini_cond.psi; ini_cond.psi_dot]
  Measurement Noise : Subsystem  TreatAsAtomicUnit=on
  Quanser AERO System Dynamics : Subsystem  TreatAsAtomicUnit=on
  Rate Transition : RateTransition  OutPortSampleTime=ts
  Rate Transition1 : RateTransition  InitialCondition=[ini_cond.theta; ini_cond.theta_dot; ini_cond.psi; ini_cond.psi_dot]  OutPortSampleTime=ts
  Selector : Selector  InputPortWidth=4  IndexOptions=Index vector (dialog)  Indices=[1 3]  OutputSizes=1
  x : Outport  VectorParamsAs1DForOutWhenUnconnected=off
  wires:
  u/1 -> Rate Transition/1
  Rate Transition/1 -> Input Noise/1(u), Demux/1
  Rate Transition1/1 -> x/1
  Input Noise/1(u_noise) -> Quanser AERO System Dynamics/2(u)
  Measurement Noise/1(x_noise) -> Rate Transition1/1
  Selector/1 -> Demux1/1
  Demux/1 -> Digital Twin/3(thruster_1)
  Demux/2 -> Digital Twin/4(thruster_2)
  Demux1/1 -> Digital Twin/1(theta)
  Demux1/2 -> Digital Twin/2(psi)
  Integrator/1 -> Measurement Noise/1(x), Selector/1, Quanser AERO System Dynamics/1(x)
  Constant/1 -> Quanser AERO System Dynamics/3(model)
  Quanser AERO System Dynamics/1(x_dot) -> Integrator/1

== system Quanser_AERO_Simulation_2020b/Quanser AERO2 ==
  u : Inport
  Constant : Constant  Value=model
  Demux : Demux  Outputs=2
  Demux1 : Demux  Outputs=2
  Digital Twin : Subsystem
  Input Noise : Subsystem  TreatAsAtomicUnit=on
  Integrator : Integrator  InitialCondition=[ini_cond.theta; ini_cond.theta_dot; ini_cond.psi; ini_cond.psi_dot]
  Measurement Noise : Subsystem  TreatAsAtomicUnit=on
  Quanser AERO System Dynamics : Subsystem  TreatAsAtomicUnit=on
  Rate Transition : RateTransition  OutPortSampleTime=ts
  Rate Transition1 : RateTransition  InitialCondition=[ini_cond.theta; ini_cond.theta_dot; ini_cond.psi; ini_cond.psi_dot]  OutPortSampleTime=ts
  Selector : Selector  InputPortWidth=4  IndexOptions=Index vector (dialog)  Indices=[1 3]  OutputSizes=1
  x : Outport  VectorParamsAs1DForOutWhenUnconnected=off
  wires:
  u/1 -> Rate Transition/1
  Rate Transition/1 -> Input Noise/1(u), Demux/1
  Rate Transition1/1 -> x/1
  Input Noise/1(u_noise) -> Quanser AERO System Dynamics/2(u)
  Measurement Noise/1(x_noise) -> Rate Transition1/1
  Selector/1 -> Demux1/1
  Demux/1 -> Digital Twin/3(thruster_1)
  Demux/2 -> Digital Twin/4(thruster_2)
  Demux1/1 -> Digital Twin/1(theta)
  Demux1/2 -> Digital Twin/2(psi)
  Integrator/1 -> Measurement Noise/1(x), Selector/1, Quanser AERO System Dynamics/1(x)
  Constant/1 -> Quanser AERO System Dynamics/3(model)
  Quanser AERO System Dynamics/1(x_dot) -> Integrator/1

== system Quanser_AERO_Simulation_2020b/Quanser AERO3 ==
  u : Inport
  Constant : Constant  Value=model
  Demux : Demux  Outputs=2
  Demux1 : Demux  Outputs=2
  Digital Twin : Subsystem
  Input Noise : Subsystem  TreatAsAtomicUnit=on
  Integrator : Integrator  InitialCondition=[ini_cond.theta; ini_cond.theta_dot; ini_cond.psi; ini_cond.psi_dot]
  Measurement Noise : Subsystem  TreatAsAtomicUnit=on
  Quanser AERO System Dynamics : Subsystem  TreatAsAtomicUnit=on
  Rate Transition : RateTransition  OutPortSampleTime=ts
  Rate Transition1 : RateTransition  InitialCondition=[ini_cond.theta; ini_cond.theta_dot; ini_cond.psi; ini_cond.psi_dot]  OutPortSampleTime=ts
  Selector : Selector  InputPortWidth=4  IndexOptions=Index vector (dialog)  Indices=[1 3]  OutputSizes=1
  x : Outport  VectorParamsAs1DForOutWhenUnconnected=off
  wires:
  u/1 -> Rate Transition/1
  Rate Transition/1 -> Input Noise/1(u), Demux/1
  Rate Transition1/1 -> x/1
  Input Noise/1(u_noise) -> Quanser AERO System Dynamics/2(u)
  Measurement Noise/1(x_noise) -> Rate Transition1/1
  Selector/1 -> Demux1/1
  Demux/1 -> Digital Twin/3(thruster_1)
  Demux/2 -> Digital Twin/4(thruster_2)
  Demux1/1 -> Digital Twin/1(theta)
  Demux1/2 -> Digital Twin/2(psi)
  Integrator/1 -> Measurement Noise/1(x), Selector/1, Quanser AERO System Dynamics/1(x)
  Constant/1 -> Quanser AERO System Dynamics/3(model)
  Quanser AERO System Dynamics/1(x_dot) -> Integrator/1

== system Quanser_AERO_Simulation_2020b/Quanser AERO4 ==
  u : Inport
  Constant : Constant  Value=model
  Demux : Demux  Outputs=2
  Demux1 : Demux  Outputs=2
  Digital Twin : Subsystem
  Input Noise : Subsystem  TreatAsAtomicUnit=on
  Integrator : Integrator  InitialCondition=[ini_cond.theta; ini_cond.theta_dot; ini_cond.psi; ini_cond.psi_dot]
  Measurement Noise : Subsystem  TreatAsAtomicUnit=on
  Quanser AERO System Dynamics : Subsystem  TreatAsAtomicUnit=on
  Rate Transition : RateTransition  OutPortSampleTime=ts
  Rate Transition1 : RateTransition  InitialCondition=[ini_cond.theta; ini_cond.theta_dot; ini_cond.psi; ini_cond.psi_dot]  OutPortSampleTime=ts
  Selector : Selector  InputPortWidth=4  IndexOptions=Index vector (dialog)  Indices=[1 3]  OutputSizes=1
  x : Outport  VectorParamsAs1DForOutWhenUnconnected=off
  wires:
  u/1 -> Rate Transition/1
  Rate Transition/1 -> Input Noise/1(u), Demux/1
  Rate Transition1/1 -> x/1
  Input Noise/1(u_noise) -> Quanser AERO System Dynamics/2(u)
  Measurement Noise/1(x_noise) -> Rate Transition1/1
  Selector/1 -> Demux1/1
  Demux/1 -> Digital Twin/3(thruster_1)
  Demux/2 -> Digital Twin/4(thruster_2)
  Demux1/1 -> Digital Twin/1(theta)
  Demux1/2 -> Digital Twin/2(psi)
  Integrator/1 -> Measurement Noise/1(x), Selector/1, Quanser AERO System Dynamics/1(x)
  Constant/1 -> Quanser AERO System Dynamics/3(model)
  Quanser AERO System Dynamics/1(x_dot) -> Integrator/1

== system Quanser_AERO_Simulation_2020b/Quanser AERO5 ==
  u : Inport
  Constant : Constant  Value=model
  Demux : Demux  Outputs=2
  Demux1 : Demux  Outputs=2
  Digital Twin : Subsystem
  Input Noise : Subsystem  TreatAsAtomicUnit=on
  Integrator : Integrator  InitialCondition=[ini_cond.theta; ini_cond.theta_dot; ini_cond.psi; ini_cond.psi_dot]
  Measurement Noise : Subsystem  TreatAsAtomicUnit=on
  Quanser AERO System Dynamics : Subsystem  TreatAsAtomicUnit=on
  Rate Transition : RateTransition  OutPortSampleTime=ts
  Rate Transition1 : RateTransition  InitialCondition=[ini_cond.theta; ini_cond.theta_dot; ini_cond.psi; ini_cond.psi_dot]  OutPortSampleTime=ts
  Selector : Selector  InputPortWidth=4  IndexOptions=Index vector (dialog)  Indices=[1 3]  OutputSizes=1
  x : Outport  VectorParamsAs1DForOutWhenUnconnected=off
  wires:
  u/1 -> Rate Transition/1
  Rate Transition/1 -> Input Noise/1(u), Demux/1
  Rate Transition1/1 -> x/1
  Input Noise/1(u_noise) -> Quanser AERO System Dynamics/2(u)
  Measurement Noise/1(x_noise) -> Rate Transition1/1
  Selector/1 -> Demux1/1
  Demux/1 -> Digital Twin/3(thruster_1)
  Demux/2 -> Digital Twin/4(thruster_2)
  Demux1/1 -> Digital Twin/1(theta)
  Demux1/2 -> Digital Twin/2(psi)
  Integrator/1 -> Measurement Noise/1(x), Selector/1, Quanser AERO System Dynamics/1(x)
  Constant/1 -> Quanser AERO System Dynamics/3(model)
  Quanser AERO System Dynamics/1(x_dot) -> Integrator/1

== system Quanser_AERO_Simulation_2020b/Quanser AERO6 ==
  u : Inport
  Constant : Constant  Value=model
  Demux : Demux  Outputs=2
  Demux1 : Demux  Outputs=2
  Digital Twin : Subsystem
  Input Noise : Subsystem  TreatAsAtomicUnit=on
  Integrator : Integrator  InitialCondition=[ini_cond.theta; ini_cond.theta_dot; ini_cond.psi; ini_cond.psi_dot]
  Measurement Noise : Subsystem  TreatAsAtomicUnit=on
  Quanser AERO System Dynamics : Subsystem  TreatAsAtomicUnit=on
  Rate Transition : RateTransition  OutPortSampleTime=ts
  Rate Transition1 : RateTransition  InitialCondition=[ini_cond.theta; ini_cond.theta_dot; ini_cond.psi; ini_cond.psi_dot]  OutPortSampleTime=ts
  Selector : Selector  InputPortWidth=4  IndexOptions=Index vector (dialog)  Indices=[1 3]  OutputSizes=1
  x : Outport  VectorParamsAs1DForOutWhenUnconnected=off
  wires:
  u/1 -> Rate Transition/1
  Rate Transition/1 -> Input Noise/1(u), Demux/1
  Rate Transition1/1 -> x/1
  Input Noise/1(u_noise) -> Quanser AERO System Dynamics/2(u)
  Measurement Noise/1(x_noise) -> Rate Transition1/1
  Selector/1 -> Demux1/1
  Demux/1 -> Digital Twin/3(thruster_1)
  Demux/2 -> Digital Twin/4(thruster_2)
  Demux1/1 -> Digital Twin/1(theta)
  Demux1/2 -> Digital Twin/2(psi)
  Integrator/1 -> Measurement Noise/1(x), Selector/1, Quanser AERO System Dynamics/1(x)
  Constant/1 -> Quanser AERO System Dynamics/3(model)
  Quanser AERO System Dynamics/1(x_dot) -> Integrator/1

== system Quanser_AERO_Simulation_2020b/Quanser AERO7 ==
  u : Inport
  Constant : Constant  Value=model
  Demux : Demux  Outputs=2
  Demux1 : Demux  Outputs=2
  Digital Twin : Subsystem
  Input Noise : Subsystem  TreatAsAtomicUnit=on
  Integrator : Integrator  InitialCondition=[ini_cond.theta; ini_cond.theta_dot; ini_cond.psi; ini_cond.psi_dot]
  Measurement Noise : Subsystem  TreatAsAtomicUnit=on
  Quanser AERO System Dynamics : Subsystem  TreatAsAtomicUnit=on
  Rate Transition : RateTransition  OutPortSampleTime=ts
  Rate Transition1 : RateTransition  InitialCondition=[ini_cond.theta; ini_cond.theta_dot; ini_cond.psi; ini_cond.psi_dot]  OutPortSampleTime=ts
  Selector : Selector  InputPortWidth=4  IndexOptions=Index vector (dialog)  Indices=[1 3]  OutputSizes=1
  x : Outport  VectorParamsAs1DForOutWhenUnconnected=off
  wires:
  u/1 -> Rate Transition/1
  Rate Transition/1 -> Input Noise/1(u), Demux/1
  Rate Transition1/1 -> x/1
  Input Noise/1(u_noise) -> Quanser AERO System Dynamics/2(u)
  Measurement Noise/1(x_noise) -> Rate Transition1/1
  Selector/1 -> Demux1/1
  Demux/1 -> Digital Twin/3(thruster_1)
  Demux/2 -> Digital Twin/4(thruster_2)
  Demux1/1 -> Digital Twin/1(theta)
  Demux1/2 -> Digital Twin/2(psi)
  Integrator/1 -> Measurement Noise/1(x), Selector/1, Quanser AERO System Dynamics/1(x)
  Constant/1 -> Quanser AERO System Dynamics/3(model)
  Quanser AERO System Dynamics/1(x_dot) -> Integrator/1

== system Quanser_AERO_Simulation_2020b/Quanser AERO8 ==
  u : Inport
  Constant : Constant  Value=model
  Demux : Demux  Outputs=2
  Demux1 : Demux  Outputs=2
  Digital Twin : Subsystem
  Input Noise : Subsystem  TreatAsAtomicUnit=on
  Integrator : Integrator  InitialCondition=[ini_cond.theta; ini_cond.theta_dot; ini_cond.psi; ini_cond.psi_dot]
  Measurement Noise : Subsystem  TreatAsAtomicUnit=on
  Quanser AERO System Dynamics : Subsystem  TreatAsAtomicUnit=on
  Rate Transition : RateTransition  OutPortSampleTime=ts
  Rate Transition1 : RateTransition  InitialCondition=[ini_cond.theta; ini_cond.theta_dot; ini_cond.psi; ini_cond.psi_dot]  OutPortSampleTime=ts
  Selector : Selector  InputPortWidth=4  IndexOptions=Index vector (dialog)  Indices=[1 3]  OutputSizes=1
  x : Outport  VectorParamsAs1DForOutWhenUnconnected=off
  wires:
  u/1 -> Rate Transition/1
  Rate Transition/1 -> Input Noise/1(u), Demux/1
  Rate Transition1/1 -> x/1
  Input Noise/1(u_noise) -> Quanser AERO System Dynamics/2(u)
  Measurement Noise/1(x_noise) -> Rate Transition1/1
  Selector/1 -> Demux1/1
  Demux/1 -> Digital Twin/3(thruster_1)
  Demux/2 -> Digital Twin/4(thruster_2)
  Demux1/1 -> Digital Twin/1(theta)
  Demux1/2 -> Digital Twin/2(psi)
  Integrator/1 -> Measurement Noise/1(x), Selector/1, Quanser AERO System Dynamics/1(x)
  Constant/1 -> Quanser AERO System Dynamics/3(model)
  Quanser AERO System Dynamics/1(x_dot) -> Integrator/1

== system Quanser_AERO_Simulation_2020b/Quanser AERO9 ==
  u : Inport
  Constant : Constant  Value=model
  Demux : Demux  Outputs=2
  Demux1 : Demux  Outputs=2
  Digital Twin : Subsystem
  Input Noise : Subsystem  TreatAsAtomicUnit=on
  Integrator : Integrator  InitialCondition=[ini_cond.theta; ini_cond.theta_dot; ini_cond.psi; ini_cond.psi_dot]
  Measurement Noise : Subsystem  TreatAsAtomicUnit=on
  Quanser AERO System Dynamics : Subsystem  TreatAsAtomicUnit=on
  Rate Transition : RateTransition  OutPortSampleTime=ts
  Rate Transition1 : RateTransition  InitialCondition=[ini_cond.theta; ini_cond.theta_dot; ini_cond.psi; ini_cond.psi_dot]  OutPortSampleTime=ts
  Selector : Selector  InputPortWidth=4  IndexOptions=Index vector (dialog)  Indices=[1 3]  OutputSizes=1
  x : Outport  VectorParamsAs1DForOutWhenUnconnected=off
  wires:
  u/1 -> Rate Transition/1
  Rate Transition/1 -> Input Noise/1(u), Demux/1
  Rate Transition1/1 -> x/1
  Input Noise/1(u_noise) -> Quanser AERO System Dynamics/2(u)
  Measurement Noise/1(x_noise) -> Rate Transition1/1
  Selector/1 -> Demux1/1
  Demux/1 -> Digital Twin/3(thruster_1)
  Demux/2 -> Digital Twin/4(thruster_2)
  Demux1/1 -> Digital Twin/1(theta)
  Demux1/2 -> Digital Twin/2(psi)
  Integrator/1 -> Measurement Noise/1(x), Selector/1, Quanser AERO System Dynamics/1(x)
  Constant/1 -> Quanser AERO System Dynamics/3(model)
  Quanser AERO System Dynamics/1(x_dot) -> Integrator/1
